simulink model "L8"  (R2012b)
settings: Solver=ode45  StartTime=0.0  StopTime=10.  MaxStep=0.05  RelTol=1e-3
libraries: simulink x2
settings Model: Creator=Артур  LastModifiedBy=Артур

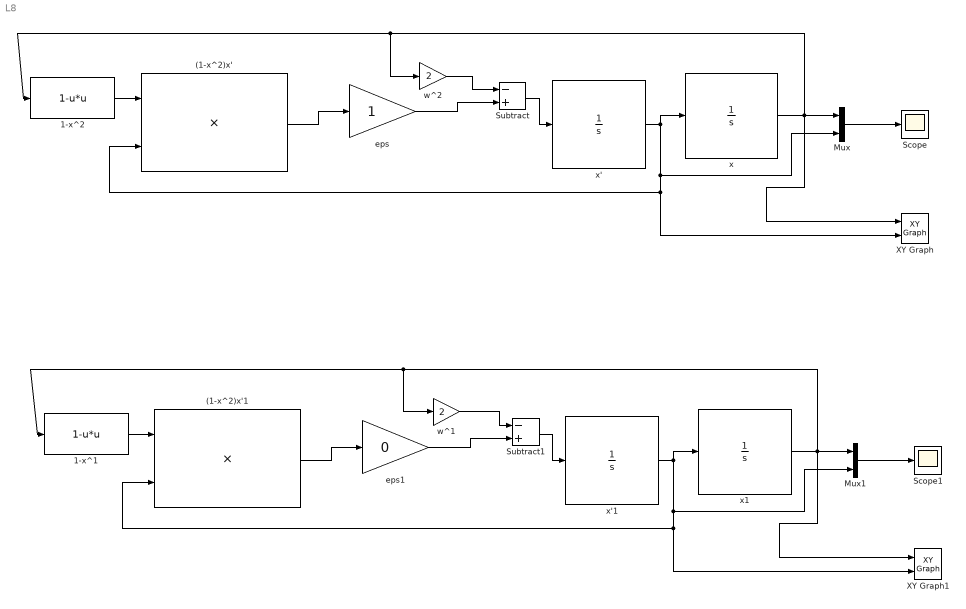
== system L8 ==
  (1-x^2)x' : Product  RndMeth=Zero
  (1-x^2)x'1 : Product  RndMeth=Zero
  1-x^1 : Fcn  Expr=1-u*u
  1-x^2 : Fcn  Expr=1-u*u
  Mux : Mux  Inputs=2
  Mux1 : Mux  Inputs=2
  Scope : Scope
  Scope1 : Scope
  Subtract : Sum  Inputs=-+
  Subtract1 : Sum  Inputs=-+
  XY Graph : simulink/Sinks/XY Graph  xmin=-1  xmax=1  ymin=-1  ymax=1  st=-1
  XY Graph1 : simulink/Sinks/XY Graph  xmin=-1  xmax=1  ymin=-1  ymax=1  st=-1
  eps : Gain
  eps1 : Gain  Gain=0
  w^1 : Gain  Gain=2
  w^2 : Gain  Gain=2
  x : Integrator  InitialCondition=0.02
  x' : Integrator  InitialCondition=0.002
  x'1 : Integrator  InitialCondition=0.002
  x1 : Integrator  InitialCondition=0.02
  wires:
  1-x^2/1 -> (1-x^2)x'/1
  x'/1 -> XY Graph/2, (1-x^2)x'/2, Mux/2, x/1
  eps/1 -> Subtract/2
  (1-x^2)x'/1 -> eps/1
  x/1 -> w^2/1, 1-x^2/1, Mux/1, XY Graph/1
  Subtract/1 -> x'/1
  Mux/1 -> Scope/1
  w^2/1 -> Subtract/1
  1-x^1/1 -> (1-x^2)x'1/1
  x'1/1 -> XY Graph1/2, (1-x^2)x'1/2, Mux1/2, x1/1
  eps1/1 -> Subtract1/2
  (1-x^2)x'1/1 -> eps1/1
  x1/1 -> w^1/1, 1-x^1/1, Mux1/1, XY Graph1/1
  Subtract1/1 -> x'1/1
  Mux1/1 -> Scope1/1
  w^1/1 -> Subtract1/1
